simulink model "Lab03S"  (R2023b)
settings: Solver=VariableStepAuto  StartTime=0.0  StopTime=1800  RelTol=1e-3
values from neighbouring files (symbols this model uses):
  A = [0 -1 5; 0 0 3; 0 0 -2]    [Lab01.m]    (also in Lab03.m = double(subs(A,x,x_eq)); Lab04.m = double(subs(A,[x u],[x_eq u_eq])); Lab05.m = [0 1; -3 -4])
  alpha = inv(-(C-D(:,1)*K)*((A-B(:,1)*K)\B(:,1))+D(:,1))    [Lab03.m]    (also in Lab04.m = inv(-C*((A-B*K)\B)); Lab05.m = inv(-C*((A-B*K)\B)); Prob1.m = 0.05; Prob2.m = 0.05)
  B = [1 1 1]'    [Lab01.m]    (also in Lab03.m = double(subs(B,u,u_eq)); Lab04.m = double(subs(B,[x u],[x_eq u_eq])); Lab05.m = [0 ; 1])
  gamma_eq = 0    [Lab03.m]
  Gb = 81    [Lab03.m]
  Ib = 15    [Lab03.m]
  K = place(A,B(:,1),lambda_k)    [Lab03.m]    (also in Lab04.m = place(A,B,lambda_k); Lab05.m = place(A,B,lambda_k))
  n = 5/54    (= 0.0925925925926)    [Lab03.m]
  p1 = 0.003    [Lab03.m]
  p2 = 0.025    [Lab03.m]
  p3 = 0.000013    (= 1.3e-05)    [Lab03.m]
  r_eq = 16.66667    [Lab03.m]
  V1 = 12    [Lab03.m]
  VG = 126    [Lab03.m]
  x_eq = double([ G_eq I_eq beta_eq ])    [Lab03.m]    (also in Lab04.m = x_eq(2,:))
libraries: simulink x4
settings Model: Creator=matteo  LastModifiedBy=matteo

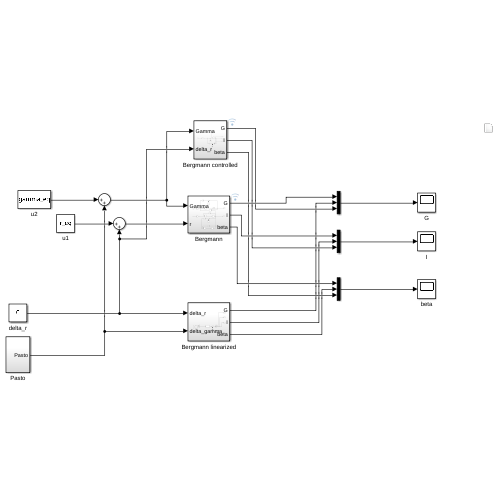
[thumbnail: Simulink's stored preview of the top-level diagram]
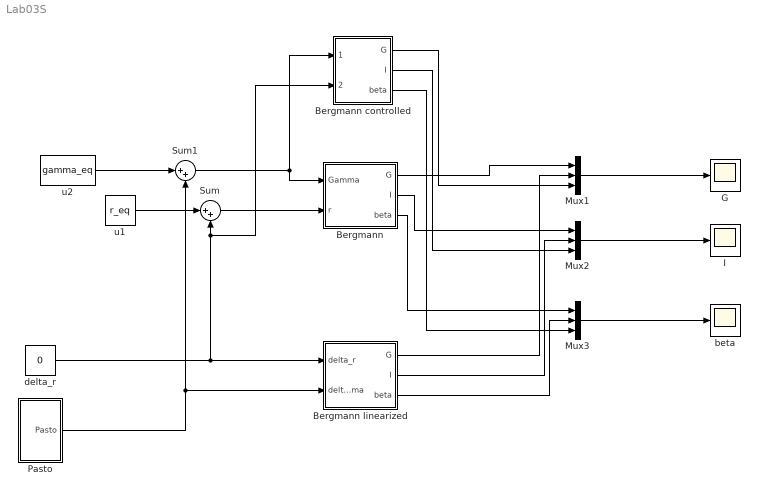
== system Lab03S ==
  Bergmann : Subsystem
  Bergmann controlled : Subsystem
  Bergmann linearized : Subsystem
  G : Scope
  I : Scope
  Mux1 : Mux  Inputs=3
  Mux2 : Mux  Inputs=3
  Mux3 : Mux  Inputs=3
  Pasto : Subsystem
  Sum : Sum  Inputs=|++
  Sum1 : Sum  Inputs=|++
  beta : Scope
  delta_r : Constant  Value=0
  u1 : Constant  Value=r_eq
  u2 : Constant  Value=gamma_eq
  wires:
  Pasto/1(Pasto) -> Sum1/2, Bergmann linearized/2(delta_gamma)
  delta_r/1 -> Bergmann linearized/1(delta_r), Bergmann controlled/2(delta_r), Sum/2
  u1/1 -> Sum/1
  Sum/1 -> Bergmann/2(r)
  u2/1 -> Sum1/1
  Sum1/1 -> Bergmann controlled/1(Gamma), Bergmann/1(Gamma)
  Mux1/1 -> G/1
  Mux2/1 -> I/1
  Mux3/1 -> beta/1
  Bergmann/1(G) -> Mux1/1
  Bergmann/2(I) -> Mux2/1
  Bergmann/3(beta) -> Mux3/1
  Bergmann controlled/1(G) -> Mux1/3
  Bergmann controlled/2(I) -> Mux2/3
  Bergmann controlled/3(beta) -> Mux3/3
  Bergmann linearized/1(G) -> Mux1/2
  Bergmann linearized/2(I) -> Mux2/2
  Bergmann linearized/3(beta) -> Mux3/2

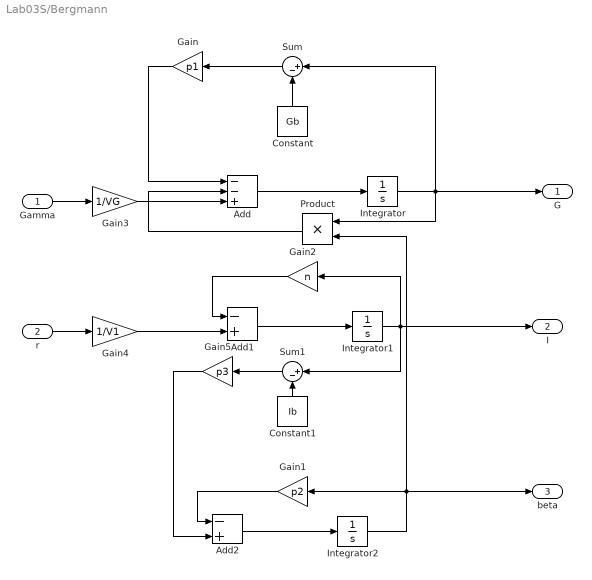
== system Lab03S/Bergmann ==
  Gamma : Inport
  r : Inport  Port=2
  Add : Sum  Inputs=--+
  Add1 : Sum  Inputs=-+
  Add2 : Sum  Inputs=-+
  Constant : Constant  Value=Gb
  Constant1 : Constant  Value=Ib
  Gain : Gain  Gain=p1
  Gain1 : Gain  Gain=p2
  Gain2 : Gain  Gain=n
  Gain3 : Gain  Gain=1/VG
  Gain4 : Gain  Gain=1/V1
  Gain5 : Gain  Gain=p3
  Integrator : Integrator  InitialCondition=x_eq(1)
  Integrator1 : Integrator  InitialCondition=x_eq(2)
  Integrator2 : Integrator  InitialCondition=x_eq(3)
  Product : Product
  Sum : Sum  Inputs=|+-
  Sum1 : Sum  Inputs=|+-
  G : Outport
  I : Outport  Port=2
  beta : Outport  Port=3
  wires:
  Gain4/1 -> Add1/2
  Gain3/1 -> Add/3
  Gamma/1 -> Gain3/1
  Add1/1 -> Integrator1/1
  Add2/1 -> Integrator2/1
  Constant/1 -> Sum/2
  Integrator2/1 -> Product/2, beta/1, Gain1/1
  Gain5/1 -> Add2/2
  Constant1/1 -> Sum1/2
  Gain2/1 -> Add1/1
  Integrator1/1 -> I/1, Sum1/1, Gain2/1
  Gain1/1 -> Add2/1
  Gain/1 -> Add/1
  Sum/1 -> Gain/1
  Integrator/1 -> G/1, Sum/1, Product/1
  Add/1 -> Integrator/1
  r/1 -> Gain4/1
  Sum1/1 -> Gain5/1
  Product/1 -> Add/2

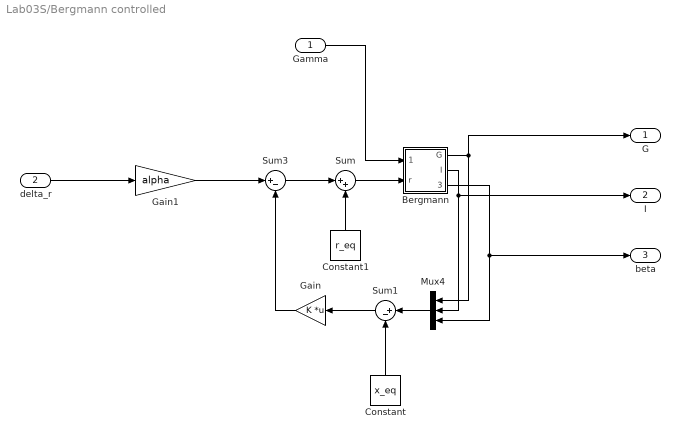
== system Lab03S/Bergmann controlled ==
  Gamma : Inport
  delta_r : Inport  Port=2
  Bergmann : Subsystem
  Constant : Constant  Value=x_eq
  Constant1 : Constant  Value=r_eq
  Gain : Gain  Gain=K  Multiplication=Matrix(K*u)
  Gain1 : Gain  Gain=alpha
  Mux4 : Mux  Inputs=3
  Sum : Sum  Inputs=|++
  Sum1 : Sum  Inputs=|+-
  Sum3 : Sum  Inputs=|+-
  G : Outport
  I : Outport  Port=2
  beta : Outport  Port=3
  wires:
  Gain/1 -> Sum3/2
  Gamma/1 -> Bergmann/1(Gamma)
  delta_r/1 -> Gain1/1
  Gain1/1 -> Sum3/1
  Bergmann/3(beta) -> beta/1, Mux4/3
  Bergmann/1(G) -> G/1, Mux4/1
  Bergmann/2(I) -> I/1, Mux4/2
  Sum3/1 -> Sum/1
  Sum/1 -> Bergmann/2(r)
  Sum1/1 -> Gain/1
  Mux4/1 -> Sum1/1
  Constant/1 -> Sum1/2
  Constant1/1 -> Sum/2

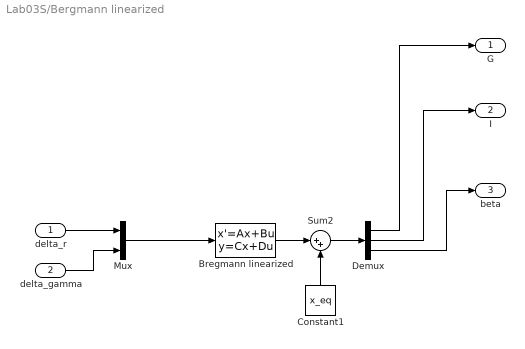
== system Lab03S/Bergmann linearized ==
  delta_r : Inport
  delta_gamma : Inport  Port=2
  Bregmann linearized : StateSpace  A=A  B=B  C=eye(3,3)  D=zeros(3,2)  InitialCondition=[9 0 0]
  Constant1 : Constant  Value=x_eq
  Demux : Demux  Outputs=3
  Mux : Mux  Inputs=2
  Sum2 : Sum  Inputs=|++
  G : Outport
  I : Outport  Port=2
  beta : Outport  Port=3
  wires:
  Sum2/1 -> Demux/1
  Bregmann linearized/1 -> Sum2/1
  Constant1/1 -> Sum2/2
  delta_gamma/1 -> Mux/2
  Mux/1 -> Bregmann linearized/1
  Demux/1 -> G/1
  Demux/3 -> beta/1
  delta_r/1 -> Mux/1
  Demux/2 -> I/1

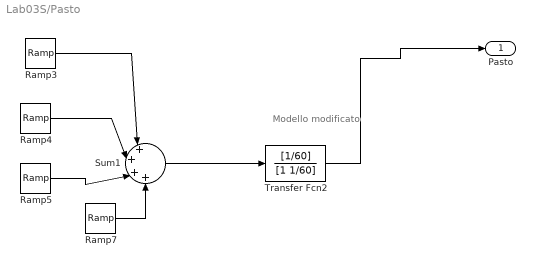
== system Lab03S/Pasto ==
  note: Modello
      | modificato
  Ramp3 : simulink/Sources/Ramp  slope=12  start=0  InitialOutput=0
  Ramp4 : simulink/Sources/Ramp  slope=-12  start=30  InitialOutput=0
  Ramp5 : simulink/Sources/Ramp  slope=-12  start=90  InitialOutput=0
  Ramp7 : simulink/Sources/Ramp  slope=12  start=120  InitialOutput=0
  Sum1 : Sum  Inputs=|+|+|+|+  InputSameDT=on  SaturateOnIntegerOverflow=on  OutDataTypeStr=Inherit: Same as first input
  Transfer Fcn2 : TransferFcn  Numerator=[1/60]  Denominator=[1 1/60]
  Pasto : Outport
  wires:
  Ramp3/1 -> Sum1/1
  Ramp4/1 -> Sum1/2
  Ramp5/1 -> Sum1/3
  Ramp7/1 -> Sum1/4
  Sum1/1 -> Transfer Fcn2/1
  Transfer Fcn2/1 -> Pasto/1

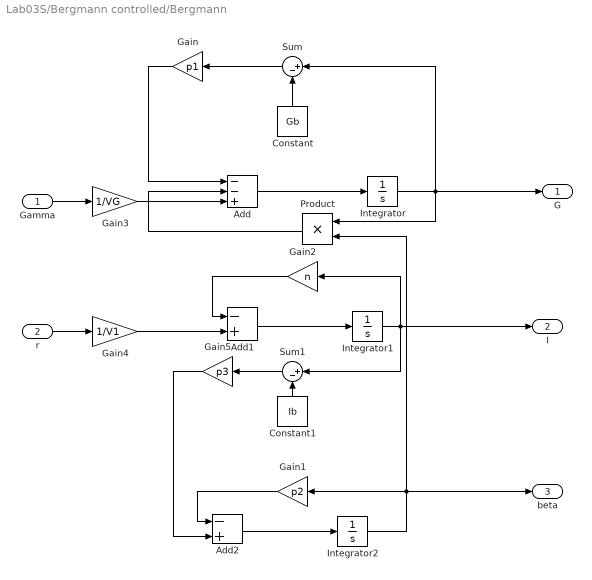
== system Lab03S/Bergmann controlled/Bergmann ==
  Gamma : Inport
  r : Inport  Port=2
  Add : Sum  Inputs=--+
  Add1 : Sum  Inputs=-+
  Add2 : Sum  Inputs=-+
  Constant : Constant  Value=Gb
  Constant1 : Constant  Value=Ib
  Gain : Gain  Gain=p1
  Gain1 : Gain  Gain=p2
  Gain2 : Gain  Gain=n
  Gain3 : Gain  Gain=1/VG
  Gain4 : Gain  Gain=1/V1
  Gain5 : Gain  Gain=p3
  Integrator : Integrator  InitialCondition=x_eq(1)
  Integrator1 : Integrator  InitialCondition=x_eq(2)
  Integrator2 : Integrator  InitialCondition=x_eq(3)
  Product : Product
  Sum : Sum  Inputs=|+-
  Sum1 : Sum  Inputs=|+-
  G : Outport
  I : Outport  Port=2
  beta : Outport  Port=3
  wires:
  Gain4/1 -> Add1/2
  Gain3/1 -> Add/3
  Gamma/1 -> Gain3/1
  Add1/1 -> Integrator1/1
  Add2/1 -> Integrator2/1
  Constant/1 -> Sum/2
  Integrator2/1 -> Product/2, beta/1, Gain1/1
  Gain5/1 -> Add2/2
  Constant1/1 -> Sum1/2
  Gain2/1 -> Add1/1
  Integrator1/1 -> I/1, Sum1/1, Gain2/1
  Gain1/1 -> Add2/1
  Gain/1 -> Add/1
  Sum/1 -> Gain/1
  Integrator/1 -> G/1, Sum/1, Product/1
  Add/1 -> Integrator/1
  r/1 -> Gain4/1
  Sum1/1 -> Gain5/1
  Product/1 -> Add/2
